simulink model "DroneControl_Sense"  (R2020a)
settings: Solver=VariableStepAuto  StartTime=0.0  StopTime=30  RelTol=1e-3
values from neighbouring files (symbols this model uses):
  body_rate_0 = [0;0;0]    [Takeoff.m]
  Boundaries = [B1;B2;B3]    [Takeoff.m]
  CMz_drone = 0-CMz    [Takeoff.m]
  CMz_tank = D_d2t + CMz    [Takeoff.m]
  Euler_0 = [0;0;0]    [Takeoff.m]
  g = [0;0;-9.8]    [Takeoff.m]
  I_Drone = [0.3933,0.3933,0.76]    [Takeoff.m]
  I_Tank = CalItank(m_tank,0.4,0.1,0.4,i)    [Takeoff.m]
  m = m_drone + m_tank*percent    (= 36)    [Takeoff.m]    (also in animation.m = T_V1toI*T_V2toV1*T_BtoV2)
  m_drone = 20    [Takeoff.m]
  m_tank = 16    [Takeoff.m]
  MaxThrust = 4*MaxMotorThrsut    (= 529.2)    [Takeoff.m]
  MaxTilt = 30*pi/180    (= 0.523598775598)    [Takeoff.m]
  MaxTorque_XY = (T2-T1)*(l/sqrt(2))    [Takeoff.m]
  MaxVel = 1.5    [Takeoff.m]
  MaxYawRate = 100*pi/180    (= 1.74532925199)    [Takeoff.m]
  percent = 1    [Takeoff.m]
  ts = 0.01    [Takeoff.m]
  WayPts = [[XYZ_0(1) XYZ_0(2) XYZ_0(3)] ... (first row only)    [Takeoff.m]
  XYZ_0 = [0;0;0]    [Takeoff.m]
undefined symbols (not defined in the file or in its folder): AccelGain, DiscIntNeverNeededParam
libraries: simulink x16, vrlib x2, aerolibutil x1
(part 1 of 2)
settings Model: NumberOfSteps=10  Creator=blaze8871  LastModifiedBy=blaze8871
settings DataIOCC: SaveTime=off

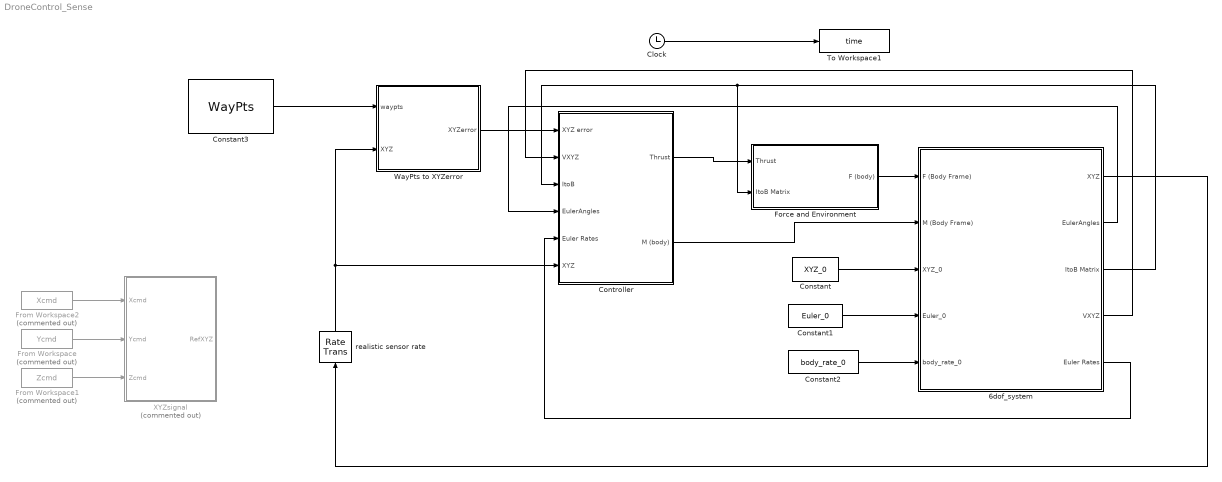
== system DroneControl_Sense ==
  6dof_system : Subsystem
  Clock : Clock
  Constant : Constant  Value=XYZ_0  SampleTime=-1
  Constant1 : Constant  Value=Euler_0  SampleTime=-1
  Constant2 : Constant  Value=body_rate_0  SampleTime=-1
  Constant3 : Constant  Value=WayPts
  Controller : Subsystem
  Force and Environment : Subsystem
  From Workspace : FromWorkspace  Commented=on  VariableName=Ycmd  SampleTime=ts
  From Workspace1 : FromWorkspace  Commented=on  VariableName=Zcmd  SampleTime=ts
  From Workspace2 : FromWorkspace  Commented=on  VariableName=Xcmd  SampleTime=ts
  To Workspace1 : ToWorkspace  VariableName=time  SampleTime=ts
  WayPts to XYZerror : MATLAB Function  TreatAsAtomicUnit=on
  XYZsignal : MATLAB Function  Commented=on  TreatAsAtomicUnit=on
  realistic sensor rate : RateTransition  OutPortSampleTime=ts
  wires:
  Constant/1 -> 6dof_system/3(XYZ_0)
  Constant1/1 -> 6dof_system/4(Euler_0)
  Constant2/1 -> 6dof_system/5(body_rate_0)
  6dof_system/1(XYZ) -> realistic sensor rate/1
  Force and Environment/1(F (body)) -> 6dof_system/1(F (Body Frame))
  6dof_system/2(EulerAngles) -> Controller/4(EulerAngles)
  WayPts to XYZerror/1(XYZerror) -> Controller/1(XYZ error)
  6dof_system/4(VXYZ) -> Controller/2(VXYZ)
  Controller/2(M (body)) -> 6dof_system/2(M (Body Frame))
  Controller/1(Thrust) -> Force and Environment/1(Thrust)
  realistic sensor rate/1 -> WayPts to XYZerror/2(XYZ), Controller/6(XYZ)
  6dof_system/5(Euler Rates) -> Controller/5(Euler Rates)
  From Workspace2/1 -> XYZsignal/1(Xcmd)
  From Workspace/1 -> XYZsignal/2(Ycmd)
  From Workspace1/1 -> XYZsignal/3(Zcmd)
  6dof_system/3(ItoB Matrix) -> Force and Environment/2(ItoB Matrix), Controller/3(ItoB)
  Constant3/1 -> WayPts to XYZerror/1(waypts)
  Clock/1 -> To Workspace1/1

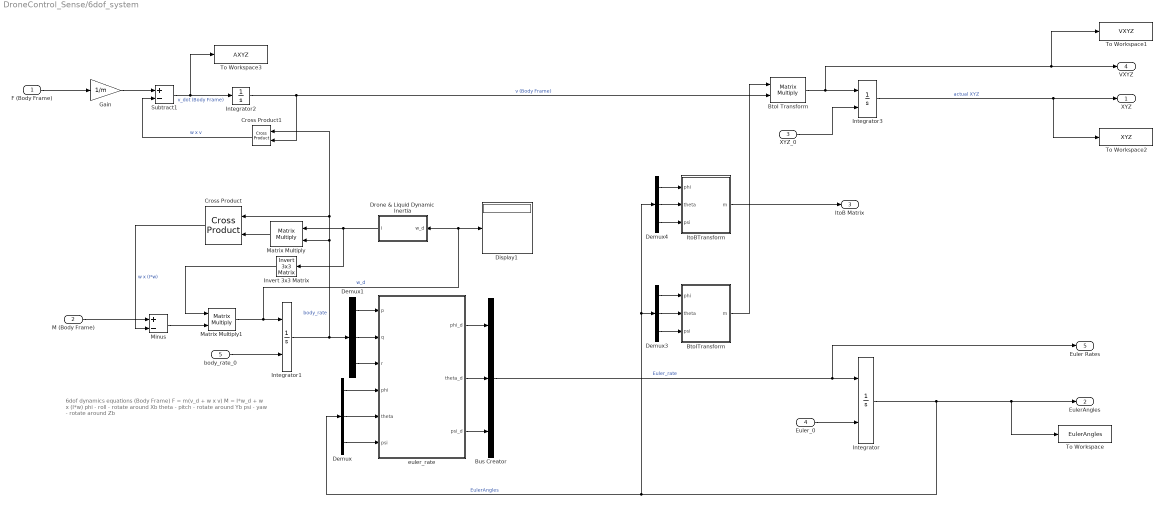
== system DroneControl_Sense/6dof_system ==
  note: 6dof dynamics equations
      | (Body Frame)
      |
      | F = m(v_d + w x v)
      | M = I*w_d + w x (I*w)
      |
      | phi - roll - rotate around Xb
      | theta - pitch - rotate around Yb
      | psi - yaw - rotate around Zb
  F (Body Frame) : Inport
  M (Body Frame) : Inport  Port=2
  XYZ_0 : Inport  Port=3
  Euler_0 : Inport  Port=4
  body_rate_0 : Inport  Port=5
  BtoI Transform : Product  Multiplication=Matrix(*)
  BtoITransform : MATLAB Function  TreatAsAtomicUnit=on
  Bus Creator : BusCreator  Inputs=3
  Cross Product : vrlib/Utilities/Cross Product
  Cross Product1 : vrlib/Utilities/Cross Product
  Demux{,1,3..4} (4 alike) : Demux  Outputs=3
  Display1 : Display
  Drone & Liquid Dynamic Inertia : Subsystem
  Gain : Gain  Gain=1/m
  Integrator : Integrator  InitialConditionSource=external  ContinuousStateAttributes='EulerAngle'
  Integrator1 : Integrator  InitialConditionSource=external  ContinuousStateAttributes='EulerAngle'
  Integrator2 : Integrator
  Integrator3 : Integrator  InitialConditionSource=external
  Invert 3x3 Matrix : aerolibutil/Invert  3x3 Matrix
  ItoBTransform : MATLAB Function  TreatAsAtomicUnit=on
  Matrix Multiply : Product  Multiplication=Matrix(*)
  Matrix Multiply1 : Product  Multiplication=Matrix(*)
  Minus : Sum  Inputs=+-
  Subtract1 : Sum  Inputs=+-
  To Workspace : ToWorkspace  VariableName=EulerAngles  SampleTime=ts
  To Workspace1 : ToWorkspace  VariableName=VXYZ  SampleTime=ts
  To Workspace2 : ToWorkspace  VariableName=XYZ  SampleTime=ts
  To Workspace3 : ToWorkspace  VariableName=AXYZ  SampleTime=ts
  euler_rate : MATLAB Function  TreatAsAtomicUnit=on
  XYZ : Outport
  EulerAngles : Outport  Port=2
  ItoB Matrix : Outport  Port=3
  VXYZ : Outport  Port=4
  Euler Rates : Outport  Port=5
  wires:
  F (Body Frame)/1 -> Gain/1
  Demux4/2 -> ItoBTransform/2(theta)
  euler_rate/1(phi_d) -> Bus Creator/1
  BtoITransform/1(m) -> BtoI Transform/1
  Bus Creator/1 -> Euler Rates/1, Integrator/1  "Euler_rate"
  Matrix Multiply/1 -> Cross Product/2
  Demux3/2 -> BtoITransform/2(theta)
  Demux/2 -> euler_rate/5(theta)
  Demux4/1 -> ItoBTransform/1(phi)
  Subtract1/1 -> To Workspace3/1, Integrator2/1  "v_dot (Body Frame)"
  Cross Product1/1 -> Subtract1/2  "w x v"
  Demux1/1 -> euler_rate/1(p)
  Demux/3 -> euler_rate/6(psi)
  euler_rate/2(theta_d) -> Bus Creator/2
  Euler_0/1 -> Integrator/2
  Integrator3/1 -> To Workspace2/1, XYZ/1  "actual XYZ"
  Cross Product/1 -> Minus/2  "w x (I*w)"
  M (Body Frame)/1 -> Minus/1
  body_rate_0/1 -> Integrator1/2
  Demux3/3 -> BtoITransform/3(psi)
  euler_rate/3(psi_d) -> Bus Creator/3
  Demux4/3 -> ItoBTransform/3(psi)
  Gain/1 -> Subtract1/1
  Demux3/1 -> BtoITransform/1(phi)
  Demux1/3 -> euler_rate/3(r)
  XYZ_0/1 -> Integrator3/2
  Demux/1 -> euler_rate/4(phi)
  Integrator2/1 -> Cross Product1/2, BtoI Transform/2  "v (Body Frame)"
  Integrator1/1 -> Cross Product1/1, Cross Product/1, Matrix Multiply/2, Demux1/1  "body_rate"
  Demux1/2 -> euler_rate/2(q)
  ItoBTransform/1(m) -> ItoB Matrix/1
  BtoI Transform/1 -> To Workspace1/1, VXYZ/1, Integrator3/1
  Minus/1 -> Matrix Multiply1/2
  Matrix Multiply1/1 -> Integrator1/1, Display1/1, Drone & Liquid Dynamic Inertia/1(w_d)  "w_d"
  Invert 3x3 Matrix/1 -> Matrix Multiply1/1
  Integrator/1 -> To Workspace/1, EulerAngles/1, Demux4/1, Demux3/1, Demux/1  "EulerAngles"
  Drone & Liquid Dynamic Inertia/1(I) -> Invert 3x3 Matrix/1, Matrix Multiply/1

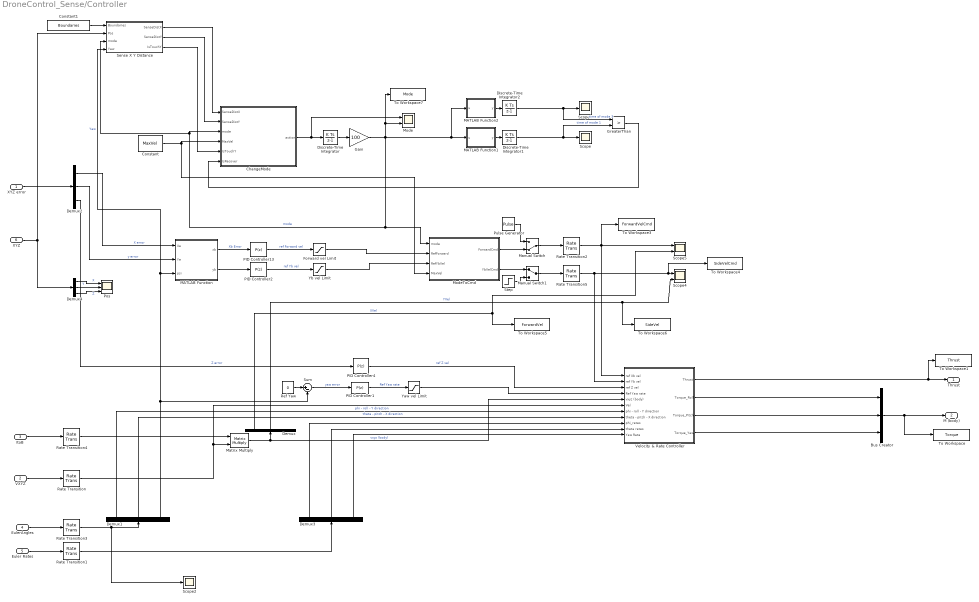
== system DroneControl_Sense/Controller ==
  XYZ error : Inport
  VXYZ : Inport  Port=2
  ItoB : Inport  Port=3
  EulerAngles : Inport  Port=4
  Euler Rates : Inport  Port=5
  XYZ : Inport  Port=6
  Bus Creator : BusCreator  Inputs=3
  ChangeMode : MATLAB Function  TreatAsAtomicUnit=on
  Constant : Constant  Value=MaxVel
  Constant1 : Constant  Value=Boundaries
  Demux{,1..4} (5 alike) : Demux  Outputs=3
  Discrete-Time Integrator : DiscreteIntegrator  SampleTime=ts  ICPrevOutput=DiscIntNeverNeededParam  ICPrevScaledInput=DiscIntNeverNeededParam
  Discrete-Time Integrator1 : DiscreteIntegrator  SampleTime=ts  ICPrevOutput=DiscIntNeverNeededParam  ICPrevScaledInput=DiscIntNeverNeededParam
  Discrete-Time Integrator2 : DiscreteIntegrator  SampleTime=ts  ICPrevOutput=DiscIntNeverNeededParam  ICPrevScaledInput=DiscIntNeverNeededParam
  Forward vel Limit : Saturate  UpperLimit=MaxVel  LowerLimit=-MaxVel
  Gain : Gain  Gain=100
  GreaterThan : RelationalOperator  Operator=>  OutDataTypeStr=boolean  RndMeth=Simplest
  MATLAB Function : MATLAB Function  TreatAsAtomicUnit=on
  MATLAB Function1 : MATLAB Function  TreatAsAtomicUnit=on
  MATLAB Function2 : MATLAB Function  TreatAsAtomicUnit=on
  Manual Switch : ManualSwitch  CurrentSetting=0
  Manual Switch1 : ManualSwitch
  Matrix Multiply : Product  Multiplication=Matrix(*)
  Mode : Scope  NumInputPorts=2
  ModeToCmd : MATLAB Function  TreatAsAtomicUnit=on
  PID Controller1 : simulink/Continuous/PID Controller  Controller=P  Form=Parallel  TimeDomain=Discrete-time  UseExternalTs=off  SampleTime=ts  IntegratorMethod=Forward Euler  FilterMethod=Forward Euler  ControllerParametersSource=internal  P=6  I=1  D=0  UseFilter=on  N=100  TunerSelectOption=Transfer Function Based (PID Tuner App)  InitialConditionSource=internal  InitialConditionForIntegrator=0  InitialConditionForFilter=0  DifferentiatorICPrevScaledInput=0  ExternalReset=none  TrackingMode=off  Kt=1  LimitOutput=off  UpperSaturationLimit=inf  LowerSaturationLimit=-inf  LinearizeAsGain=on  AntiWindupMode=none  Kb=1  POutMin=[]  POutMax=[]  IOutMin=[]  IOutMax=[]  DOutMin=[]  DOutMax=[]  NOutMin=[]  NOutMax=[]  SumOutMin=[]  SumOutMax=[]  SaturationOutMin=[]  SaturationOutMax=[]  PParamMin=[]  PParamMax=[]  IParamMin=[]  IParamMax=[]  DParamMin=[]  DParamMax=[]  NParamMin=[]  NParamMax=[]  KbParamMin=[]  KbParamMax=[]  KtParamMin=[]  KtParamMax=[]  KbOutMin=[]  KbOutMax=[]  KtOutMin=[]  KtOutMax=[]  IntegratorOutMin=[]  IntegratorOutMax=[]  FilterOutMin=[]  FilterOutMax=[]  SumI1OutMin=[]  SumI1OutMax=[]  SumI2OutMin=[]  SumI2OutMax=[]  SumI3OutMin=[]  SumI3OutMax=[]  SumI4OutMin=[]  SumI4OutMax=[]  SumDOutMin=[]  SumDOutMax=[]  DifferentiatorOutMin=[]  DifferentiatorOutMax=[]  FilterDiffOutCoefMin=[]  FilterDiffOutCoefMax=[]  ReciprocalOutMin=[]  ReciprocalOutMax=[]  SumDenOutMin=[]  SumDenOutMax=[]  SumNumOutMin=[]  SumNumOutMax=[]  DivideOutMin=[]  DivideOutMax=[]  UdiffTsProdOutMin=[]  UdiffTsProdOutMax=[]  NTsProdOutMin=[]  NTsProdOutMax=[]  UintegralTsProdOutMin=[]  UintegralTsProdOutMax=[]  UngainTsProdOutMin=[]  UngainTsProdOutMax=[]  IntegratorContinuousStateAttributes=''  IntegratorStateMustResolveToSignalObject=off  IntegratorRTWStateStorageClass=Auto  FilterContinuousStateAttributes=''  FilterStateMustResolveToSignalObject=off  FilterRTWStateStorageClass=Auto  ParallelPVariant=InternalParameters  IdealPVariant=Disabled  IVariant=Disabled  DVariant=Disabled  IntegratorVariant=Disabled  SatVariant=Disabled  AWVariant=Disabled  PCopyVariant=Disabled  TRVariant=Disabled  FdbkBlocksVariant=Forward  IdealPFdbkVariant=Disabled  SatFdbkVariant=Disabled  DerivativeFilterVariant=Disabled  NVariant=Disabled  NCopyVariant=Disabled_SignalSpec  FilterICVariant=Disabled  IntegratorICVariant=Disabled  ExternalResetVariant=Disabled  TRSumVariant=Passthrough  SumFdbkVariant=Disabled  SumVariant=Passthrough_P  TsampFilterVariant=InternalTs  TsampNgainVariant=Passthrough  TsampIntegralVariant=Disabled_SignalSpec
  PID Controller13 : simulink/Continuous/PID Controller  Controller=P  Form=Parallel  TimeDomain=Discrete-time  UseExternalTs=off  SampleTime=ts  IntegratorMethod=Forward Euler  FilterMethod=Forward Euler  ControllerParametersSource=internal  P=0.6  I=1  D=0  UseFilter=on  N=100  TunerSelectOption=Transfer Function Based (PID Tuner App)  InitialConditionSource=internal  InitialConditionForIntegrator=0  InitialConditionForFilter=0  DifferentiatorICPrevScaledInput=0  ExternalReset=none  TrackingMode=off  Kt=1  LimitOutput=off  UpperSaturationLimit=inf  LowerSaturationLimit=-inf  LinearizeAsGain=on  AntiWindupMode=none  Kb=1  POutMin=[]  POutMax=[]  IOutMin=[]  IOutMax=[]  DOutMin=[]  DOutMax=[]  NOutMin=[]  NOutMax=[]  SumOutMin=[]  SumOutMax=[]  SaturationOutMin=[]  SaturationOutMax=[]  PParamMin=[]  PParamMax=[]  IParamMin=[]  IParamMax=[]  DParamMin=[]  DParamMax=[]  NParamMin=[]  NParamMax=[]  KbParamMin=[]  KbParamMax=[]  KtParamMin=[]  KtParamMax=[]  KbOutMin=[]  KbOutMax=[]  KtOutMin=[]  KtOutMax=[]  IntegratorOutMin=[]  IntegratorOutMax=[]  FilterOutMin=[]  FilterOutMax=[]  SumI1OutMin=[]  SumI1OutMax=[]  SumI2OutMin=[]  SumI2OutMax=[]  SumI3OutMin=[]  SumI3OutMax=[]  SumI4OutMin=[]  SumI4OutMax=[]  SumDOutMin=[]  SumDOutMax=[]  DifferentiatorOutMin=[]  DifferentiatorOutMax=[]  FilterDiffOutCoefMin=[]  FilterDiffOutCoefMax=[]  ReciprocalOutMin=[]  ReciprocalOutMax=[]  SumDenOutMin=[]  SumDenOutMax=[]  SumNumOutMin=[]  SumNumOutMax=[]  DivideOutMin=[]  DivideOutMax=[]  UdiffTsProdOutMin=[]  UdiffTsProdOutMax=[]  NTsProdOutMin=[]  NTsProdOutMax=[]  UintegralTsProdOutMin=[]  UintegralTsProdOutMax=[]  UngainTsProdOutMin=[]  UngainTsProdOutMax=[]  IntegratorContinuousStateAttributes=''  IntegratorStateMustResolveToSignalObject=off  IntegratorRTWStateStorageClass=Auto  FilterContinuousStateAttributes=''  FilterStateMustResolveToSignalObject=off  FilterRTWStateStorageClass=Auto  ParallelPVariant=InternalParameters  IdealPVariant=Disabled  IVariant=Disabled  DVariant=Disabled  IntegratorVariant=Disabled  SatVariant=Disabled  AWVariant=Disabled  PCopyVariant=Disabled  TRVariant=Disabled  FdbkBlocksVariant=Forward  IdealPFdbkVariant=Disabled  SatFdbkVariant=Disabled  DerivativeFilterVariant=Disabled  NVariant=Disabled  NCopyVariant=Disabled_SignalSpec  FilterICVariant=Disabled  IntegratorICVariant=Disabled  ExternalResetVariant=Disabled  TRSumVariant=Passthrough  SumFdbkVariant=Disabled  SumVariant=Passthrough_P  TsampFilterVariant=InternalTs  TsampNgainVariant=Passthrough  TsampIntegralVariant=Disabled_SignalSpec
  PID Controller2 : simulink/Continuous/PID Controller  Controller=P  Form=Parallel  TimeDomain=Discrete-time  UseExternalTs=off  SampleTime=ts  IntegratorMethod=Forward Euler  FilterMethod=Forward Euler  ControllerParametersSource=internal  P=0.6  I=1  D=0  UseFilter=on  N=100  TunerSelectOption=Transfer Function Based (PID Tuner App)  InitialConditionSource=internal  InitialConditionForIntegrator=0  InitialConditionForFilter=0  DifferentiatorICPrevScaledInput=0  ExternalReset=none  TrackingMode=off  Kt=1  LimitOutput=off  UpperSaturationLimit=inf  LowerSaturationLimit=-inf  LinearizeAsGain=on  AntiWindupMode=none  Kb=1  POutMin=[]  POutMax=[]  IOutMin=[]  IOutMax=[]  DOutMin=[]  DOutMax=[]  NOutMin=[]  NOutMax=[]  SumOutMin=[]  SumOutMax=[]  SaturationOutMin=[]  SaturationOutMax=[]  PParamMin=[]  PParamMax=[]  IParamMin=[]  IParamMax=[]  DParamMin=[]  DParamMax=[]  NParamMin=[]  NParamMax=[]  KbParamMin=[]  KbParamMax=[]  KtParamMin=[]  KtParamMax=[]  KbOutMin=[]  KbOutMax=[]  KtOutMin=[]  KtOutMax=[]  IntegratorOutMin=[]  IntegratorOutMax=[]  FilterOutMin=[]  FilterOutMax=[]  SumI1OutMin=[]  SumI1OutMax=[]  SumI2OutMin=[]  SumI2OutMax=[]  SumI3OutMin=[]  SumI3OutMax=[]  SumI4OutMin=[]  SumI4OutMax=[]  SumDOutMin=[]  SumDOutMax=[]  DifferentiatorOutMin=[]  DifferentiatorOutMax=[]  FilterDiffOutCoefMin=[]  FilterDiffOutCoefMax=[]  ReciprocalOutMin=[]  ReciprocalOutMax=[]  SumDenOutMin=[]  SumDenOutMax=[]  SumNumOutMin=[]  SumNumOutMax=[]  DivideOutMin=[]  DivideOutMax=[]  UdiffTsProdOutMin=[]  UdiffTsProdOutMax=[]  NTsProdOutMin=[]  NTsProdOutMax=[]  UintegralTsProdOutMin=[]  UintegralTsProdOutMax=[]  UngainTsProdOutMin=[]  UngainTsProdOutMax=[]  IntegratorContinuousStateAttributes=''  IntegratorStateMustResolveToSignalObject=off  IntegratorRTWStateStorageClass=Auto  FilterContinuousStateAttributes=''  FilterStateMustResolveToSignalObject=off  FilterRTWStateStorageClass=Auto  ParallelPVariant=InternalParameters  IdealPVariant=Disabled  IVariant=Disabled  DVariant=Disabled  IntegratorVariant=Disabled  SatVariant=Disabled  AWVariant=Disabled  PCopyVariant=Disabled  TRVariant=Disabled  FdbkBlocksVariant=Forward  IdealPFdbkVariant=Disabled  SatFdbkVariant=Disabled  DerivativeFilterVariant=Disabled  NVariant=Disabled  NCopyVariant=Disabled_SignalSpec  FilterICVariant=Disabled  IntegratorICVariant=Disabled  ExternalResetVariant=Disabled  TRSumVariant=Passthrough  SumFdbkVariant=Disabled  SumVariant=Passthrough_P  TsampFilterVariant=InternalTs  TsampNgainVariant=Passthrough  TsampIntegralVariant=Disabled_SignalSpec
  PID Controller4 : simulink/Continuous/PID Controller  Controller=P  Form=Parallel  TimeDomain=Discrete-time  UseExternalTs=off  SampleTime=ts  IntegratorMethod=Forward Euler  FilterMethod=Forward Euler  ControllerParametersSource=internal  P=2.48254445381199  I=1  D=0  UseFilter=on  N=100  TunerSelectOption=Transfer Function Based (PID Tuner App)  InitialConditionSource=internal  InitialConditionForIntegrator=0  InitialConditionForFilter=0  DifferentiatorICPrevScaledInput=0  ExternalReset=none  TrackingMode=off  Kt=1  LimitOutput=off  UpperSaturationLimit=inf  LowerSaturationLimit=-inf  LinearizeAsGain=on  AntiWindupMode=none  Kb=1  POutMin=[]  POutMax=[]  IOutMin=[]  IOutMax=[]  DOutMin=[]  DOutMax=[]  NOutMin=[]  NOutMax=[]  SumOutMin=[]  SumOutMax=[]  SaturationOutMin=[]  SaturationOutMax=[]  PParamMin=[]  PParamMax=[]  IParamMin=[]  IParamMax=[]  DParamMin=[]  DParamMax=[]  NParamMin=[]  NParamMax=[]  KbParamMin=[]  KbParamMax=[]  KtParamMin=[]  KtParamMax=[]  KbOutMin=[]  KbOutMax=[]  KtOutMin=[]  KtOutMax=[]  IntegratorOutMin=[]  IntegratorOutMax=[]  FilterOutMin=[]  FilterOutMax=[]  SumI1OutMin=[]  SumI1OutMax=[]  SumI2OutMin=[]  SumI2OutMax=[]  SumI3OutMin=[]  SumI3OutMax=[]  SumI4OutMin=[]  SumI4OutMax=[]  SumDOutMin=[]  SumDOutMax=[]  DifferentiatorOutMin=[]  DifferentiatorOutMax=[]  FilterDiffOutCoefMin=[]  FilterDiffOutCoefMax=[]  ReciprocalOutMin=[]  ReciprocalOutMax=[]  SumDenOutMin=[]  SumDenOutMax=[]  SumNumOutMin=[]  SumNumOutMax=[]  DivideOutMin=[]  DivideOutMax=[]  UdiffTsProdOutMin=[]  UdiffTsProdOutMax=[]  NTsProdOutMin=[]  NTsProdOutMax=[]  UintegralTsProdOutMin=[]  UintegralTsProdOutMax=[]  UngainTsProdOutMin=[]  UngainTsProdOutMax=[]  IntegratorContinuousStateAttributes=''  IntegratorStateMustResolveToSignalObject=off  IntegratorRTWStateStorageClass=Auto  FilterContinuousStateAttributes=''  FilterStateMustResolveToSignalObject=off  FilterRTWStateStorageClass=Auto  ParallelPVariant=InternalParameters  IdealPVariant=Disabled  IVariant=Disabled  DVariant=Disabled  IntegratorVariant=Disabled  SatVariant=Disabled  AWVariant=Disabled  PCopyVariant=Disabled  TRVariant=Disabled  FdbkBlocksVariant=Forward  IdealPFdbkVariant=Disabled  SatFdbkVariant=Disabled  DerivativeFilterVariant=Disabled  NVariant=Disabled  NCopyVariant=Disabled_SignalSpec  FilterICVariant=Disabled  IntegratorICVariant=Disabled  ExternalResetVariant=Disabled  TRSumVariant=Passthrough  SumFdbkVariant=Disabled  SumVariant=Passthrough_P  TsampFilterVariant=InternalTs  TsampNgainVariant=Passthrough  TsampIntegralVariant=Disabled_SignalSpec
  Pos : Scope  NumInputPorts=3
  Pulse Generator : DiscretePulseGenerator  PulseType=Time based  Period=20  PulseWidth=25  PhaseDelay=1
  Rate Transition{,1..5} (6 alike) : RateTransition  OutPortSampleTime=ts
  Ref Yaw : Constant  Value=0
  Scope : Scope
  Scope1 : Scope
  Scope2 : Scope
  Scope4 : Scope  NumInputPorts=2
  Scope5 : Scope  NumInputPorts=2
  Sense X Y Distance : Subsystem
  Step : Step  After=0  SampleTime=0
  Sum : Sum  Inputs=|+-
  To Workspace : ToWorkspace  VariableName=Torque  SampleTime=ts
  To Workspace1 : ToWorkspace  VariableName=Thrust  SampleTime=ts
  To Workspace3 : ToWorkspace  VariableName=ForwardVelCmd  SampleTime=ts
  To Workspace4 : ToWorkspace  VariableName=SideVelCmd  SampleTime=ts
  To Workspace5 : ToWorkspace  VariableName=ForwardVel  SampleTime=ts
  To Workspace6 : ToWorkspace  VariableName=SideVel  SampleTime=ts
  To Workspace7 : ToWorkspace  VariableName=Mode  SampleTime=ts
  Velocity & Rate Controller : Subsystem
  Yaw vel Limit : Saturate  UpperLimit=MaxYawRate  LowerLimit=-MaxYawRate
  Yb vel Limit : Saturate  UpperLimit=MaxVel  LowerLimit=-MaxVel
  Thrust : Outport
  M (body) : Outport  Port=2
  wires:
  Bus Creator/1 -> To Workspace/1, M (body)/1
  VXYZ/1 -> Rate Transition/1
  Demux2/3 -> PID Controller4/1  "Z error"
  EulerAngles/1 -> Rate Transition3/1
  Demux1/3 -> MATLAB Function/3(psi), Sense X Y Distance/4(Yaw), Sum/2  "Yaw"
  Sum/1 -> PID Controller1/1  "yaw error"
  ItoB/1 -> Rate Transition4/1
  XYZ error/1 -> Demux2/1
  Rate Transition3/1 -> Scope2/1, Demux1/1
  Rate Transition4/1 -> Matrix Multiply/1
  Euler Rates/1 -> Rate Transition1/1
  Rate Transition1/1 -> Demux3/1
  Demux2/1 -> MATLAB Function/1(Xe)  "X error"
  Demux2/2 -> MATLAB Function/2(Ye)  "y error"
  Rate Transition/1 -> Velocity & Rate Controller/6(Vel), Matrix Multiply/2
  MATLAB Function/1(xb) -> PID Controller13/1  "Xb Error"
  PID Controller13/1 -> Forward vel Limit/1  "ref Forward vel"
  Matrix Multiply/1 -> Velocity & Rate Controller/5(vxyz (body)), Demux/1  "vxyz (body)"
  PID Controller4/1 -> Velocity & Rate Controller/3(ref Z vel)  "ref Z vel"
  PID Controller1/1 -> Yaw vel Limit/1  "Ref Yaw rate"
  Demux1/1 -> Velocity & Rate Controller/7(phi - roll - Y direction)  "phi - roll - Y direction"
  Demux1/2 -> Velocity & Rate Controller/8(theta - pitch - X direction)  "theta - pitch - X direction"
  Demux3/1 -> Velocity & Rate Controller/9(phi_rates)
  Demux3/2 -> Velocity & Rate Controller/10(theta rates)
  Demux3/3 -> Velocity & Rate Controller/11(Yaw Rate)
  Velocity & Rate Controller/1(Thrust) -> To Workspace1/1, Thrust/1
  Velocity & Rate Controller/2(Torque_Roll) -> Bus Creator/1
  Velocity & Rate Controller/3(Torque_Pitch) -> Bus Creator/2
  Velocity & Rate Controller/4(Torque_Yaw) -> Bus Creator/3
  Forward vel Limit/1 -> ModeToCmd/2(RefForward)
  Yaw vel Limit/1 -> Velocity & Rate Controller/4(Ref Yaw rate)
  Ref Yaw/1 -> Sum/1
  MATLAB Function/2(yb) -> PID Controller2/1
  PID Controller2/1 -> Yb vel Limit/1  "ref Yb vel"
  Yb vel Limit/1 -> ModeToCmd/3(RefYbVel)
  XYZ/1 -> Sense X Y Distance/2(Pos), Demux4/1
  Demux4/1 -> Pos/1  "X"
  Demux4/2 -> Pos/2  "Y"
  Demux4/3 -> Pos/3  "Z"
  ChangeMode/1(action) -> Mode/1, Discrete-Time Integrator/1
  Discrete-Time Integrator/1 -> Gain/1
  Gain/1 -> To Workspace7/1, Mode/2, Sense X Y Distance/3(mode), ChangeMode/3(mode), ModeToCmd/1(mode), MATLAB Function2/1(u), MATLAB Function1/1(u)  "mode"
  Constant/1 -> ModeToCmd/4(MaxVel), ChangeMode/4(MaxVel)
  Manual Switch1/1 -> Rate Transition5/1
  Demux/2 -> To Workspace6/1, Scope4/2  "YVel"
  Demux/1 -> To Workspace5/1, Scope5/2  "XVel"
  Pulse Generator/1 -> Manual Switch/1
  ModeToCmd/1(ForwardCmd) -> Manual Switch/2
  Manual Switch/1 -> Rate Transition2/1
  Step/1 -> Manual Switch1/2
  ModeToCmd/2(YbVelCmd) -> Manual Switch1/1
  Rate Transition2/1 -> To Workspace3/1, Scope5/1, Velocity & Rate Controller/1(ref Xb vel)
  Rate Transition5/1 -> To Workspace4/1, Scope4/1, Velocity & Rate Controller/2(ref Yb vel)
  Sense X Y Distance/1(SenseDistX) -> ChangeMode/1(SenseDistX)
  Constant1/1 -> Sense X Y Distance/1(Boundaries)
  Sense X Y Distance/2(SenseDistY) -> ChangeMode/2(SenseDistY)
  Sense X Y Distance/3(IsTouchY) -> ChangeMode/5(IsTouchY)
  MATLAB Function1/1(y) -> Discrete-Time Integrator1/1
  Discrete-Time Integrator1/1 -> GreaterThan/2, Scope/1  "time of mode 1"
  Discrete-Time Integrator2/1 -> GreaterThan/1, Scope1/1  "time of mode 3"
  MATLAB Function2/1(y) -> Discrete-Time Integrator2/1
  GreaterThan/1 -> ChangeMode/6(IsRecover)

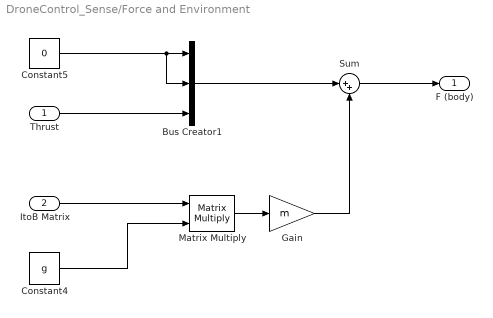
== system DroneControl_Sense/Force and Environment ==
  Thrust : Inport
  ItoB Matrix : Inport  Port=2
  Bus Creator1 : BusCreator  Inputs=3
  Constant4 : Constant  Value=g  SampleTime=-1
  Constant5 : Constant  Value=0  SampleTime=-1
  Gain : Gain  Gain=m
  Matrix Multiply : Product  Multiplication=Matrix(*)
  Sum : Sum  Inputs=|++
  F (body) : Outport
  wires:
  Thrust/1 -> Bus Creator1/3
  Bus Creator1/1 -> Sum/1
  Constant4/1 -> Matrix Multiply/2
  ItoB Matrix/1 -> Matrix Multiply/1
  Constant5/1 -> Bus Creator1/2, Bus Creator1/1
  Matrix Multiply/1 -> Gain/1
  Sum/1 -> F (body)/1
  Gain/1 -> Sum/2

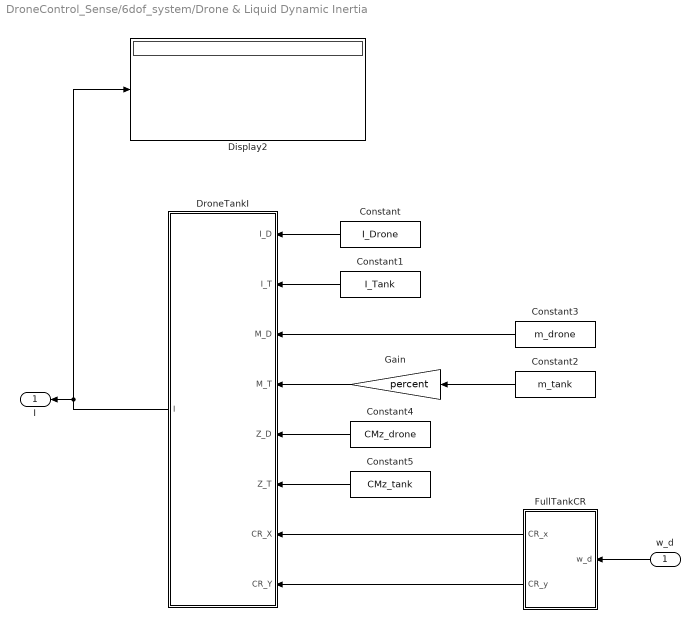
== system DroneControl_Sense/6dof_system/Drone & Liquid Dynamic Inertia ==
  w_d : Inport
  Constant : Constant  Value=I_Drone
  Constant1 : Constant  Value=I_Tank
  Constant2 : Constant  Value=m_tank
  Constant3 : Constant  Value=m_drone
  Constant4 : Constant  Value=CMz_drone
  Constant5 : Constant  Value=CMz_tank
  Display2 : Display
  DroneTankI : MATLAB Function  TreatAsAtomicUnit=on
  FullTankCR : MATLAB Function  TreatAsAtomicUnit=on
  Gain : Gain  Gain=percent
  I : Outport
  wires:
  FullTankCR/2(CR_y) -> DroneTankI/8(CR_Y)
  Constant/1 -> DroneTankI/1(I_D)
  w_d/1 -> FullTankCR/1(w_d)
  DroneTankI/1(I) -> Display2/1, I/1
  Constant1/1 -> DroneTankI/2(I_T)
  FullTankCR/1(CR_x) -> DroneTankI/7(CR_X)
  Constant3/1 -> DroneTankI/3(M_D)
  Gain/1 -> DroneTankI/4(M_T)
  Constant2/1 -> Gain/1
  Constant4/1 -> DroneTankI/5(Z_D)
  Constant5/1 -> DroneTankI/6(Z_T)

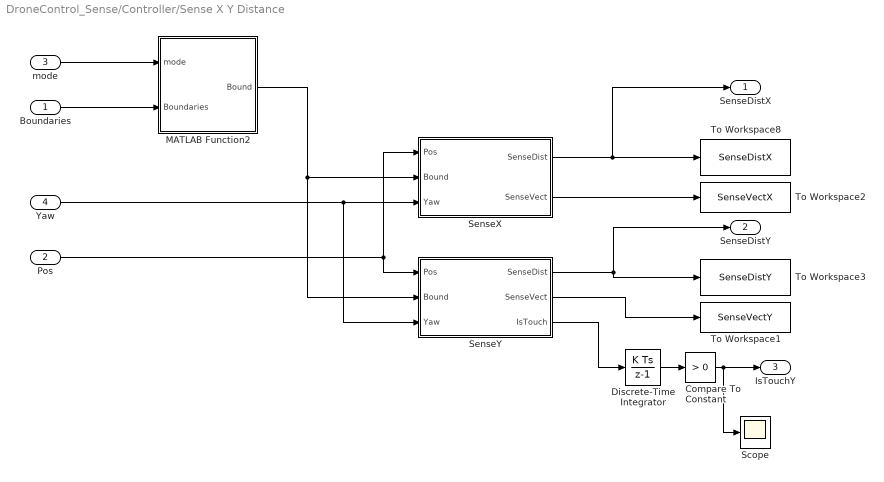
== system DroneControl_Sense/Controller/Sense X Y Distance ==
  Boundaries : Inport
  Pos : Inport  Port=2
  mode : Inport  Port=3
  Yaw : Inport  Port=4
  Compare To Constant : simulink/Logic and Bit Operations/Compare To Constant  relop=>  const=0  OutDataTypeStr=boolean
  Discrete-Time Integrator : DiscreteIntegrator  SampleTime=ts  ICPrevOutput=DiscIntNeverNeededParam  ICPrevScaledInput=DiscIntNeverNeededParam
  MATLAB Function2 : MATLAB Function  TreatAsAtomicUnit=on
  Scope : Scope
  SenseX : MATLAB Function  TreatAsAtomicUnit=on
  SenseY : MATLAB Function  TreatAsAtomicUnit=on
  To Workspace1 : ToWorkspace  VariableName=SenseVectY  SampleTime=ts
  To Workspace2 : ToWorkspace  VariableName=SenseVectX  SampleTime=ts
  To Workspace3 : ToWorkspace  VariableName=SenseDistY  SampleTime=ts
  To Workspace8 : ToWorkspace  VariableName=SenseDistX  SampleTime=ts
  SenseDistX : Outport
  SenseDistY : Outport  Port=2
  IsTouchY : Outport  Port=3
  wires:
  mode/1 -> MATLAB Function2/1(mode)
  Boundaries/1 -> MATLAB Function2/2(Boundaries)
  SenseX/2(SenseVect) -> To Workspace2/1
  SenseX/1(SenseDist) -> SenseDistX/1, To Workspace8/1
  MATLAB Function2/1(Bound) -> SenseX/2(Bound), SenseY/2(Bound)
  Yaw/1 -> SenseX/3(Yaw), SenseY/3(Yaw)
  Pos/1 -> SenseY/1(Pos), SenseX/1(Pos)
  SenseY/2(SenseVect) -> To Workspace1/1
  SenseY/1(SenseDist) -> To Workspace3/1, SenseDistY/1
  SenseY/3(IsTouch) -> Discrete-Time Integrator/1
  Discrete-Time Integrator/1 -> Compare To Constant/1
  Compare To Constant/1 -> IsTouchY/1, Scope/1

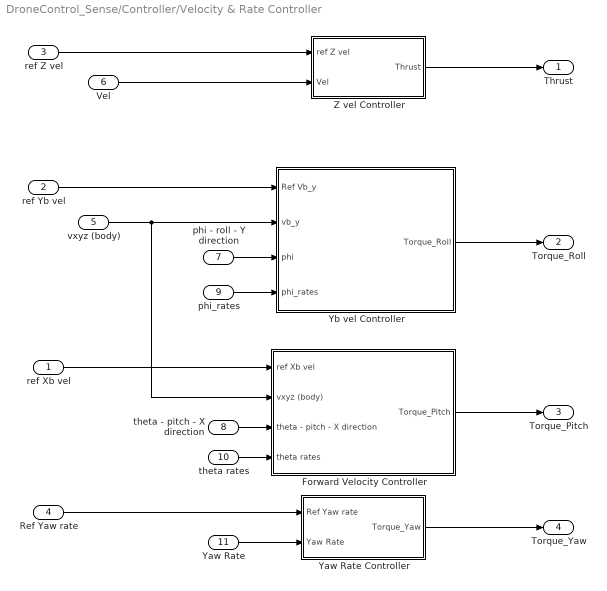
== system DroneControl_Sense/Controller/Velocity & Rate Controller ==
  ref Xb vel : Inport
  ref Yb vel : Inport  Port=2
  ref Z vel : Inport  Port=3
  Ref Yaw rate : Inport  Port=4
  vxyz (body) : Inport  Port=5
  Vel : Inport  Port=6
  phi - roll - Y direction : Inport  Port=7
  theta - pitch - X direction : Inport  Port=8
  phi_rates : Inport  Port=9
  theta rates : Inport  Port=10
  Yaw Rate : Inport  Port=11
  Forward Velocity Controller : Subsystem
  Yaw Rate Controller : Subsystem
  Yb vel Controller : Subsystem
  Z vel Controller : Subsystem
  Thrust : Outport
  Torque_Roll : Outport  Port=2
  Torque_Pitch : Outport  Port=3
  Torque_Yaw : Outport  Port=4
  wires:
  Yb vel Controller/1(Torque_Roll) -> Torque_Roll/1
  Forward Velocity Controller/1(Torque_Pitch) -> Torque_Pitch/1
  theta - pitch - X direction/1 -> Forward Velocity Controller/3(theta - pitch - X direction)
  Z vel Controller/1(Thrust) -> Thrust/1
  phi - roll - Y direction/1 -> Yb vel Controller/3(phi)
  Ref Yaw rate/1 -> Yaw Rate Controller/1(Ref Yaw rate)
  ref Z vel/1 -> Z vel Controller/1(ref Z vel)
  vxyz (body)/1 -> Yb vel Controller/2(vb_y), Forward Velocity Controller/2(vxyz (body))
  Vel/1 -> Z vel Controller/2(Vel)
  theta rates/1 -> Forward Velocity Controller/4(theta rates)
  phi_rates/1 -> Yb vel Controller/4(phi_rates)
  Yaw Rate/1 -> Yaw Rate Controller/2(Yaw Rate)
  ref Xb vel/1 -> Forward Velocity Controller/1(ref Xb vel)
  Yaw Rate Controller/1(Torque_Yaw) -> Torque_Yaw/1
  ref Yb vel/1 -> Yb vel Controller/1(Ref Vb_y)

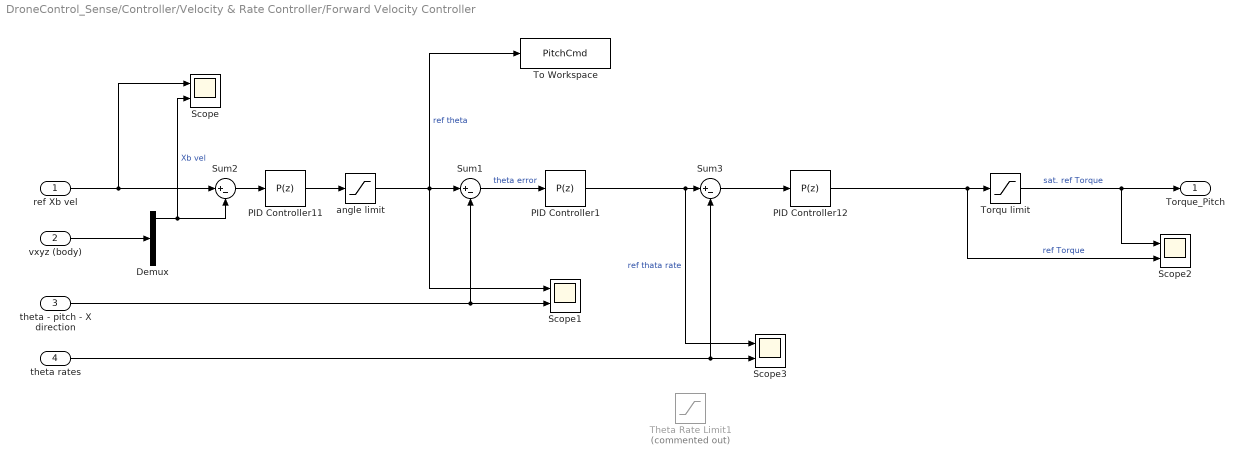
== system DroneControl_Sense/Controller/Velocity & Rate Controller/Forward Velocity Controller ==
  ref Xb vel : Inport
  vxyz (body) : Inport  Port=2
  theta - pitch - X direction : Inport  Port=3
  theta rates : Inport  Port=4
  Demux : Demux  Outputs=3
  PID Controller1 : simulink/Continuous/PID Controller  Controller=P  Form=Parallel  TimeDomain=Discrete-time  UseExternalTs=off  SampleTime=ts  IntegratorMethod=Forward Euler  FilterMethod=Forward Euler  ControllerParametersSource=internal  P=6  I=1  D=0  UseFilter=on  N=100  TunerSelectOption=Transfer Function Based (PID Tuner App)  InitialConditionSource=internal  InitialConditionForIntegrator=0  InitialConditionForFilter=0  DifferentiatorICPrevScaledInput=0  ExternalReset=none  TrackingMode=off  Kt=1  LimitOutput=off  UpperSaturationLimit=inf  LowerSaturationLimit=-inf  LinearizeAsGain=on  AntiWindupMode=none  Kb=1  POutMin=[]  POutMax=[]  IOutMin=[]  IOutMax=[]  DOutMin=[]  DOutMax=[]  NOutMin=[]  NOutMax=[]  SumOutMin=[]  SumOutMax=[]  SaturationOutMin=[]  SaturationOutMax=[]  PParamMin=[]  PParamMax=[]  IParamMin=[]  IParamMax=[]  DParamMin=[]  DParamMax=[]  NParamMin=[]  NParamMax=[]  KbParamMin=[]  KbParamMax=[]  KtParamMin=[]  KtParamMax=[]  KbOutMin=[]  KbOutMax=[]  KtOutMin=[]  KtOutMax=[]  IntegratorOutMin=[]  IntegratorOutMax=[]  FilterOutMin=[]  FilterOutMax=[]  SumI1OutMin=[]  SumI1OutMax=[]  SumI2OutMin=[]  SumI2OutMax=[]  SumI3OutMin=[]  SumI3OutMax=[]  SumI4OutMin=[]  SumI4OutMax=[]  SumDOutMin=[]  SumDOutMax=[]  DifferentiatorOutMin=[]  DifferentiatorOutMax=[]  FilterDiffOutCoefMin=[]  FilterDiffOutCoefMax=[]  ReciprocalOutMin=[]  ReciprocalOutMax=[]  SumDenOutMin=[]  SumDenOutMax=[]  SumNumOutMin=[]  SumNumOutMax=[]  DivideOutMin=[]  DivideOutMax=[]  UdiffTsProdOutMin=[]  UdiffTsProdOutMax=[]  NTsProdOutMin=[]  NTsProdOutMax=[]  UintegralTsProdOutMin=[]  UintegralTsProdOutMax=[]  UngainTsProdOutMin=[]  UngainTsProdOutMax=[]  IntegratorContinuousStateAttributes=''  IntegratorStateMustResolveToSignalObject=off  IntegratorRTWStateStorageClass=Auto  FilterContinuousStateAttributes=''  FilterStateMustResolveToSignalObject=off  FilterRTWStateStorageClass=Auto  ParallelPVariant=InternalParameters  IdealPVariant=Disabled  IVariant=Disabled  DVariant=Disabled  IntegratorVariant=Disabled  SatVariant=Disabled  AWVariant=Disabled  PCopyVariant=Disabled  TRVariant=Disabled  FdbkBlocksVariant=Forward  IdealPFdbkVariant=Disabled  SatFdbkVariant=Disabled  DerivativeFilterVariant=Disabled  NVariant=Disabled  NCopyVariant=Disabled_SignalSpec  FilterICVariant=Disabled  IntegratorICVariant=Disabled  ExternalResetVariant=Disabled  TRSumVariant=Passthrough  SumFdbkVariant=Disabled  SumVariant=Passthrough_P  TsampFilterVariant=InternalTs  TsampNgainVariant=Passthrough  TsampIntegralVariant=Disabled_SignalSpec
  PID Controller11 : simulink/Continuous/PID Controller  Controller=P  Form=Parallel  TimeDomain=Discrete-time  UseExternalTs=off  SampleTime=ts  IntegratorMethod=Forward Euler  FilterMethod=Forward Euler  ControllerParametersSource=internal  P=AccelGain  I=1  D=0  UseFilter=on  N=100  TunerSelectOption=Transfer Function Based (PID Tuner App)  InitialConditionSource=internal  InitialConditionForIntegrator=0  InitialConditionForFilter=0  DifferentiatorICPrevScaledInput=0  ExternalReset=none  TrackingMode=off  Kt=1  LimitOutput=off  UpperSaturationLimit=inf  LowerSaturationLimit=-inf  LinearizeAsGain=on  AntiWindupMode=none  Kb=1  POutMin=[]  POutMax=[]  IOutMin=[]  IOutMax=[]  DOutMin=[]  DOutMax=[]  NOutMin=[]  NOutMax=[]  SumOutMin=[]  SumOutMax=[]  SaturationOutMin=[]  SaturationOutMax=[]  PParamMin=[]  PParamMax=[]  IParamMin=[]  IParamMax=[]  DParamMin=[]  DParamMax=[]  NParamMin=[]  NParamMax=[]  KbParamMin=[]  KbParamMax=[]  KtParamMin=[]  KtParamMax=[]  KbOutMin=[]  KbOutMax=[]  KtOutMin=[]  KtOutMax=[]  IntegratorOutMin=[]  IntegratorOutMax=[]  FilterOutMin=[]  FilterOutMax=[]  SumI1OutMin=[]  SumI1OutMax=[]  SumI2OutMin=[]  SumI2OutMax=[]  SumI3OutMin=[]  SumI3OutMax=[]  SumI4OutMin=[]  SumI4OutMax=[]  SumDOutMin=[]  SumDOutMax=[]  DifferentiatorOutMin=[]  DifferentiatorOutMax=[]  FilterDiffOutCoefMin=[]  FilterDiffOutCoefMax=[]  ReciprocalOutMin=[]  ReciprocalOutMax=[]  SumDenOutMin=[]  SumDenOutMax=[]  SumNumOutMin=[]  SumNumOutMax=[]  DivideOutMin=[]  DivideOutMax=[]  UdiffTsProdOutMin=[]  UdiffTsProdOutMax=[]  NTsProdOutMin=[]  NTsProdOutMax=[]  UintegralTsProdOutMin=[]  UintegralTsProdOutMax=[]  UngainTsProdOutMin=[]  UngainTsProdOutMax=[]  IntegratorContinuousStateAttributes=''  IntegratorStateMustResolveToSignalObject=off  IntegratorRTWStateStorageClass=Auto  FilterContinuousStateAttributes=''  FilterStateMustResolveToSignalObject=off  FilterRTWStateStorageClass=Auto  ParallelPVariant=InternalParameters  IdealPVariant=Disabled  IVariant=Disabled  DVariant=Disabled  IntegratorVariant=Disabled  SatVariant=Disabled  AWVariant=Disabled  PCopyVariant=Disabled  TRVariant=Disabled  FdbkBlocksVariant=Forward  IdealPFdbkVariant=Disabled  SatFdbkVariant=Disabled  DerivativeFilterVariant=Disabled  NVariant=Disabled  NCopyVariant=Disabled_SignalSpec  FilterICVariant=Disabled  IntegratorICVariant=Disabled  ExternalResetVariant=Disabled  TRSumVariant=Passthrough  SumFdbkVariant=Disabled  SumVariant=Passthrough_P  TsampFilterVariant=InternalTs  TsampNgainVariant=Passthrough  TsampIntegralVariant=Disabled_SignalSpec
  PID Controller12 : simulink/Continuous/PID Controller  Controller=P  Form=Parallel  TimeDomain=Discrete-time  UseExternalTs=off  SampleTime=ts  IntegratorMethod=Forward Euler  FilterMethod=Forward Euler  ControllerParametersSource=internal  P=10  I=1  D=0  UseFilter=on  N=100  TunerSelectOption=Transfer Function Based (PID Tuner App)  InitialConditionSource=internal  InitialConditionForIntegrator=0  InitialConditionForFilter=0  DifferentiatorICPrevScaledInput=0  ExternalReset=none  TrackingMode=off  Kt=1  LimitOutput=off  UpperSaturationLimit=inf  LowerSaturationLimit=-inf  LinearizeAsGain=on  AntiWindupMode=none  Kb=1  POutMin=[]  POutMax=[]  IOutMin=[]  IOutMax=[]  DOutMin=[]  DOutMax=[]  NOutMin=[]  NOutMax=[]  SumOutMin=[]  SumOutMax=[]  SaturationOutMin=[]  SaturationOutMax=[]  PParamMin=[]  PParamMax=[]  IParamMin=[]  IParamMax=[]  DParamMin=[]  DParamMax=[]  NParamMin=[]  NParamMax=[]  KbParamMin=[]  KbParamMax=[]  KtParamMin=[]  KtParamMax=[]  KbOutMin=[]  KbOutMax=[]  KtOutMin=[]  KtOutMax=[]  IntegratorOutMin=[]  IntegratorOutMax=[]  FilterOutMin=[]  FilterOutMax=[]  SumI1OutMin=[]  SumI1OutMax=[]  SumI2OutMin=[]  SumI2OutMax=[]  SumI3OutMin=[]  SumI3OutMax=[]  SumI4OutMin=[]  SumI4OutMax=[]  SumDOutMin=[]  SumDOutMax=[]  DifferentiatorOutMin=[]  DifferentiatorOutMax=[]  FilterDiffOutCoefMin=[]  FilterDiffOutCoefMax=[]  ReciprocalOutMin=[]  ReciprocalOutMax=[]  SumDenOutMin=[]  SumDenOutMax=[]  SumNumOutMin=[]  SumNumOutMax=[]  DivideOutMin=[]  DivideOutMax=[]  UdiffTsProdOutMin=[]  UdiffTsProdOutMax=[]  NTsProdOutMin=[]  NTsProdOutMax=[]  UintegralTsProdOutMin=[]  UintegralTsProdOutMax=[]  UngainTsProdOutMin=[]  UngainTsProdOutMax=[]  IntegratorContinuousStateAttributes=''  IntegratorStateMustResolveToSignalObject=off  IntegratorRTWStateStorageClass=Auto  FilterContinuousStateAttributes=''  FilterStateMustResolveToSignalObject=off  FilterRTWStateStorageClass=Auto  ParallelPVariant=InternalParameters  IdealPVariant=Disabled  IVariant=Disabled  DVariant=Disabled  IntegratorVariant=Disabled  SatVariant=Disabled  AWVariant=Disabled  PCopyVariant=Disabled  TRVariant=Disabled  FdbkBlocksVariant=Forward  IdealPFdbkVariant=Disabled  SatFdbkVariant=Disabled  DerivativeFilterVariant=Disabled  NVariant=Disabled  NCopyVariant=Disabled_SignalSpec  FilterICVariant=Disabled  IntegratorICVariant=Disabled  ExternalResetVariant=Disabled  TRSumVariant=Passthrough  SumFdbkVariant=Disabled  SumVariant=Passthrough_P  TsampFilterVariant=InternalTs  TsampNgainVariant=Passthrough  TsampIntegralVariant=Disabled_SignalSpec
  Scope{,1..3} (4 alike) : Scope  NumInputPorts=2
  Sum1 : Sum  Inputs=|+-
  Sum2 : Sum  Inputs=|+-
  Sum3 : Sum  Inputs=|+-
  Theta Rate Limit1 : Saturate  Commented=on
  To Workspace : ToWorkspace  VariableName=PitchCmd  SampleTime=ts
  Torqu limit : Saturate  UpperLimit=MaxTorque_XY  LowerLimit=-MaxTorque_XY
  angle limit : Saturate  UpperLimit=MaxTilt  LowerLimit=-MaxTilt
  Torque_Pitch : Outport
  wires:
  Sum1/1 -> PID Controller1/1  "theta error"
  Demux/1 -> Scope/2, Sum2/2  "Xb vel"
  angle limit/1 -> To Workspace/1, Scope1/1, Sum1/1  "ref theta"
  Sum2/1 -> PID Controller11/1
  vxyz (body)/1 -> Demux/1
  PID Controller1/1 -> Scope3/1, Sum3/1  "ref thata rate"
  PID Controller12/1 -> Torqu limit/1, Scope2/2  "ref Torque"
  theta - pitch - X direction/1 -> Sum1/2, Scope1/2
  theta rates/1 -> Sum3/2, Scope3/2
  ref Xb vel/1 -> Scope/1, Sum2/1
  PID Controller11/1 -> angle limit/1
  Sum3/1 -> PID Controller12/1
  Torqu limit/1 -> Torque_Pitch/1, Scope2/1  "sat. ref Torque"

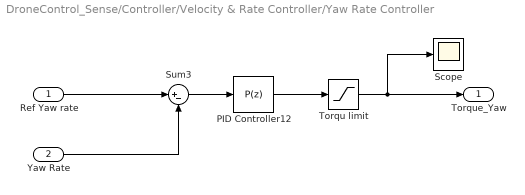
== system DroneControl_Sense/Controller/Velocity & Rate Controller/Yaw Rate Controller ==
  Ref Yaw rate : Inport
  Yaw Rate : Inport  Port=2
  PID Controller12 : simulink/Continuous/PID Controller  Controller=P  Form=Parallel  TimeDomain=Discrete-time  UseExternalTs=off  SampleTime=ts  IntegratorMethod=Forward Euler  FilterMethod=Forward Euler  ControllerParametersSource=internal  P=2  I=1  D=0  UseFilter=on  N=100  TunerSelectOption=Transfer Function Based (PID Tuner App)  InitialConditionSource=internal  InitialConditionForIntegrator=0  InitialConditionForFilter=0  DifferentiatorICPrevScaledInput=0  ExternalReset=none  TrackingMode=off  Kt=1  LimitOutput=off  UpperSaturationLimit=inf  LowerSaturationLimit=-inf  LinearizeAsGain=on  AntiWindupMode=none  Kb=1  POutMin=[]  POutMax=[]  IOutMin=[]  IOutMax=[]  DOutMin=[]  DOutMax=[]  NOutMin=[]  NOutMax=[]  SumOutMin=[]  SumOutMax=[]  SaturationOutMin=[]  SaturationOutMax=[]  PParamMin=[]  PParamMax=[]  IParamMin=[]  IParamMax=[]  DParamMin=[]  DParamMax=[]  NParamMin=[]  NParamMax=[]  KbParamMin=[]  KbParamMax=[]  KtParamMin=[]  KtParamMax=[]  KbOutMin=[]  KbOutMax=[]  KtOutMin=[]  KtOutMax=[]  IntegratorOutMin=[]  IntegratorOutMax=[]  FilterOutMin=[]  FilterOutMax=[]  SumI1OutMin=[]  SumI1OutMax=[]  SumI2OutMin=[]  SumI2OutMax=[]  SumI3OutMin=[]  SumI3OutMax=[]  SumI4OutMin=[]  SumI4OutMax=[]  SumDOutMin=[]  SumDOutMax=[]  DifferentiatorOutMin=[]  DifferentiatorOutMax=[]  FilterDiffOutCoefMin=[]  FilterDiffOutCoefMax=[]  ReciprocalOutMin=[]  ReciprocalOutMax=[]  SumDenOutMin=[]  SumDenOutMax=[]  SumNumOutMin=[]  SumNumOutMax=[]  DivideOutMin=[]  DivideOutMax=[]  UdiffTsProdOutMin=[]  UdiffTsProdOutMax=[]  NTsProdOutMin=[]  NTsProdOutMax=[]  UintegralTsProdOutMin=[]  UintegralTsProdOutMax=[]  UngainTsProdOutMin=[]  UngainTsProdOutMax=[]  IntegratorContinuousStateAttributes=''  IntegratorStateMustResolveToSignalObject=off  IntegratorRTWStateStorageClass=Auto  FilterContinuousStateAttributes=''  FilterStateMustResolveToSignalObject=off  FilterRTWStateStorageClass=Auto  ParallelPVariant=InternalParameters  IdealPVariant=Disabled  IVariant=Disabled  DVariant=Disabled  IntegratorVariant=Disabled  SatVariant=Disabled  AWVariant=Disabled  PCopyVariant=Disabled  TRVariant=Disabled  FdbkBlocksVariant=Forward  IdealPFdbkVariant=Disabled  SatFdbkVariant=Disabled  DerivativeFilterVariant=Disabled  NVariant=Disabled  NCopyVariant=Disabled_SignalSpec  FilterICVariant=Disabled  IntegratorICVariant=Disabled  ExternalResetVariant=Disabled  TRSumVariant=Passthrough  SumFdbkVariant=Disabled  SumVariant=Passthrough_P  TsampFilterVariant=InternalTs  TsampNgainVariant=Passthrough  TsampIntegralVariant=Disabled_SignalSpec
  Scope : Scope
  Sum3 : Sum  Inputs=|+-
  Torqu limit : Saturate  UpperLimit=MaxTorque_XY  LowerLimit=-MaxTorque_XY
  Torque_Yaw : Outport
  wires:
  Sum3/1 -> PID Controller12/1
  Yaw Rate/1 -> Sum3/2
  Ref Yaw rate/1 -> Sum3/1
  Torqu limit/1 -> Scope/1, Torque_Yaw/1
  PID Controller12/1 -> Torqu limit/1
